simulink model "LFPCaseStudy_ZahidSarigol"  (R2025b)
settings: Solver=VariableStepAuto  StartTime=0.0  StopTime=3600  RelTol=1e-3
libraries: fl_lib x5, nesl_utility x3, batt_lib x1
settings Model: Creator=zahid  LastModifiedBy=zahid

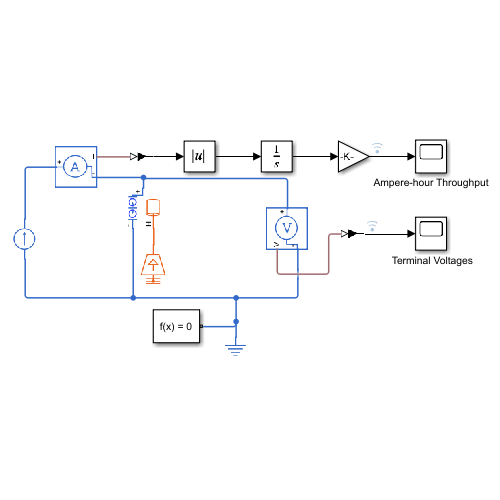
[thumbnail: Simulink's stored preview of the top-level diagram]
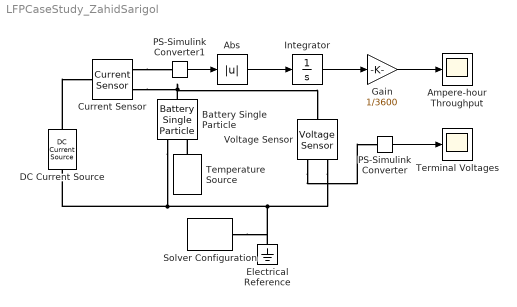
== system LFPCaseStudy_ZahidSarigol ==
  " Terminal Voltages" : Scope
      settings: ActiveDisplayYMinimum=2.7369582029139718  ActiveDisplayYMaximum=3.8258448981690734  YLabel=Voltage (V)
  Abs : Abs  SaturateOnIntegerOverflow=off
  Ampere-hour Throughput : Scope
      settings: ActiveDisplayYMinimum=-0.26295274335598895  ActiveDisplayYMaximum=2.3665746902039011  YLabel=Capacity (Ah)
  Battery Single Particle : batt_lib/Cells/Electrochemical/Battery Single Particle  ExtrapolationMethod=simscape.enum.extrapolation.nearest  ThicknessAnode=3.4E-5 m  ElectrolyteLayerCountAnode=10  ThicknessSeparator=2.5E-5 m  ElectrolyteLayerCountSeparator=5  ThicknessCathode=8E-5 m  ElectrolyteLayerCountCathode=10  ElectrodePlateArea=1.738E-1 m^2  ParticleRadiusAnode=3.5E-6 m  ShellCountAnode=10  ParticleRadiusCathode=5.2E-8 m  ShellCountCathode=10  ActiveMaterialVolumeFractionAnode=0.56  ActiveMaterialVolumeFractionCathode=0.454  StoichiometryBreakpointsSpecification=simscape.battery.enum.cells.electrochemical.StoichiometryBreakpointsSpecification.normalized  NormalizedStoichiometryBreakpoints=linspace(0.025, 0.975, 39)  OpenCircuitPotentialAnode=[.484; .335; .253; .209; .2; .181; .165; .151; .139; .131; .128; .125; .124; .124; .123; .122; .119; .117; .111; .108; .101; .098; .095; .093; .092; .088; .088; .088; .088; .087; .087; .087; .085; .082; .079; .071; .064; .049; .026] V  OpenCircuitPotentialCathode=[3.81;3.608;3.512;3.478;3.459;3.453;3.45257;3.45214;3.45171;3.45128;3.45085;3.45042;3.44999;3.44956;3.44913;3.4487;3.44827;3.44784;3.44741;3.44698;3.44655;3.44612;3.44569;3.44526;3.44483;3.4444;3.44397;3.44354;3.44311;3.44268;3.44225;3.44182;3.44139;3.44096;3.44053;3.44;3.412;3.304;2.968] V  AbsoluteStoichiometryBreakpointsAnode=linspace(0.025, 0.975, 39)  OpenCircuitPotentialAbsoluteAnode=[.484; .335; .253; .209; .2; .181; .165; .151; .139; .131; .128; .125; .124; .124; .123; .122; .119; .117; .111; .108; .101; .098; .095; .093; .092; .088; .088; .088; .088; .087; .087; .087; .085; .082; .079; .071; .064; .049; .026] V  AbsoluteStoichiometryBreakpointsCathode=linspace(0.025, 0.975, 39)  OpenCircuitPotentialAbsoluteCathode=[3.81; 3.608; 3.512; 3.478; 3.459; 3.453; 3.45257; 3.45214; 3.45171; 3.45128; 3.45085; 3.45042; 3.44999; 3.44956; 3.44913; 3.4487; 3.44827; 3.44784; 3.44741; 3.44698; 3.44655; 3.44612; 3.44569; 3.44526; 3.44483; 3.4444; 3.44397; 3.44354; 3.44311; 3.44268; 3.44225; 3.44182; 3.44139; 3.44096; 3.44053; 3.44; 3.412; 3.304; 2.968] V  MaximumConcentrationAnode=31900 mol/m^3  MaximumStoichiometryAnode=0.811  MinimumStoichiometryAnode=0.0132  MaximumConcentrationCathode=20950 mol/m^3  MaximumStoichiometryCathode=0.74  MinimumStoichiometryCathode=0.035  ActiveMaterialDiffusionCoefficientAnode=3E-15 m^2/s  ActiveMaterialDiffusionCoefficientCathode=8E-18 m^2/s  ConductivityAnode=200 S/m  ConductivityCathode=0.1 S/m  CurrentCollectorResistance=0 Ohm  ElectrolyteVolumeFractionAnode=0.3874  ElectrolyteVolumeFractionSeparator=0.45  ElectrolyteVolumeFractionCathode=0.5725  ElectrolyteConductivity=0.29 S/m  BruggemanExponentAnode=1.5  BruggemanExponentSeparator=1.5  BruggemanExponentCathode=1.5  TransferenceNumber=0.363  ElectrolyteDiffusionCoefficient=2E-10 m^2/s  ChargeTransferRateAnode=8.8E-11 m^(5/2)/(mol^(1/2)*s)  ChargeTransferRateCathode=2.8E-13 m^(5/2)/(mol^(1/2)*s)  BatteryThermalMass=77 J/K  ArrheniusReferenceTemperature=298.15 K  ActiveMaterialDiffusionActivationEnergyAnode=39000 J/mol  ActiveMaterialDiffusionActivationEnergyCathode=35000 J/mol  ElectrolyteDiffusionActivationEnergy=26600 J/mol  ConductivityActivationEnergyAnode=3000 J/mol  ConductivityActivationEnergyCathode=3000 J/mol  ElectrolyteConductivityActivationEnergy=11000 J/mol  ChargeTransferActivationEnergyAnode=13000 J/mol  ChargeTransferActivationEnergyCathode=20000 J/mol  batteryCurrent_specify=off  batteryCurrent_priority=None  batteryCurrent=0 A  batteryCurrent_nominal_specify=off  batteryCurrent_nominal_value=1  batteryCurrent_nominal_unit=A  batteryVoltage_specify=off  batteryVoltage_priority=None  batteryVoltage=0 V  batteryVoltage_nominal_specify=off  batteryVoltage_nominal_value=1  batteryVoltage_nominal_unit=V  averageElectrolyteConcentration_specify=off  averageElectrolyteConcentration_priority=High  averageElectrolyteConcentration=1200 mol/m^3  averageElectrolyteConcentration_nominal_specify=off  averageElectrolyteConcentration_nominal_value=1  averageElectrolyteConcentration_nominal_unit=mol/m^3  stateOfCharge_specify=on  stateOfCharge_priority=High  stateOfCharge=1  stateOfCharge_nominal_specify=off  stateOfCharge_nominal_value=1  stateOfCharge_nominal_unit=1  batteryTemperature_specify=off  batteryTemperature_priority=High  batteryTemperature=298.15 K  batteryTemperature_nominal_specify=off  batteryTemperature_nominal_value=1  batteryTemperature_nominal_unit=K  power_dissipated_specify=off  power_dissipated_priority=None  power_dissipated=0 W  power_dissipated_nominal_specify=off  power_dissipated_nominal_value=1  power_dissipated_nominal_unit=W  heatGenerationRate_specify=off  heatGenerationRate_priority=None  heatGenerationRate=0 W  heatGenerationRate_nominal_specify=off  heatGenerationRate_nominal_value=1  heatGenerationRate_nominal_unit=W
      settings: InternalSimscapePortConfiguration="{\"Bottom\":[],\"Left\":[{\"id\":\"p\",\"label\":\"+\",\"type\":\"foundation.electrical.electrical\"}],\"Right\":[{\"id\":\"n\",\"label\":\"-\",\"type\":\"foundation.electrical.electrical\"},{\"id\":\"H\",\"label\":\"H\",\"type\":\"foundation.thermal.thermal\"}],\"Top\":[]}"
  Current Sensor : fl_lib/Electrical/Electrical Sensors/Current Sensor
  DC Current Source : fl_lib/Electrical/Electrical Sources/DC Current Source  i0=-2.5 A
      settings: InternalSimscapePortConfiguration="{\"Bottom\":[],\"Left\":[{\"id\":\"p\",\"label\":\"\",\"type\":\"foundation.electrical.electrical\"}],\"Right\":[{\"id\":\"n\",\"label\":\"\",\"type\":\"foundation.electrical.electrical\"}],\"Top\":[]}"
  Electrical Reference : fl_lib/Electrical/Electrical Elements/Electrical Reference
  Gain : Gain  Gain=1/3600
  Integrator : Integrator
  PS-Simulink Converter : nesl_utility/PS-Simulink Converter  PhysicalDomain=network_engine_domain  SubClassName=ps_output  LeftPortType=input  RightPortType=output  PseudoPeriodic=off  Frequencies=[]  VectorFormat=inherit  Unit=inherit  AffineConversion=off
  PS-Simulink Converter1 : nesl_utility/PS-Simulink Converter  PhysicalDomain=network_engine_domain  SubClassName=ps_output  LeftPortType=input  RightPortType=output  PseudoPeriodic=off  Frequencies=[]  VectorFormat=inherit  Unit=inherit  AffineConversion=off
  Solver Configuration : nesl_utility/Solver Configuration  PhysicalDomain=network_engine_domain  SubClassName=solver  LeftPortType=input  RightPortType=generic  Tones=[]  Harmonics=[]  SimulateNoise=off  Profile=off  UseLocalSampling=off  EnableSwitchedLinearOptims=on  FrequencyDomain=off  UseCCode=off  RelTol=0.001  AbsTol=0.001  MinStep=1e-09  ToWorkspace=off  RevertToSquareIcSolve=off  NumHomotopyIterations=100  PhasorMode=off  PhasorModeNumHarmonics=1  ConsistencySolver=NEWTON_XTOL_AFTER_FTOL  IndexReductionMethod=DerivativeReplacement  DoDC=off  ResidualTolerance=1e-09  ConsistencyTolSource=GLOBAL  ConsistencyAbsTol=0.001  ConsistencyRelTol=0.001  ConsistencyTolFactor=0.001  UseLocalSolver=off  LocalSolverChoice=NE_BACKWARD_EULER_ADVANCER  ResolveIndetEquations=on  FunctionEvalNumThread=1  LocalSolverSampleTime=0.001  DoFixedCost=off  MaxNonlinIter=3  MaxModeIter=2  ComputeImpulses=off  ImpulseIterations=2  LinearAlgebra=auto  LinearAlgebraNumThread=0  EquationFormulation=NE_TIME_EF  DelaysMemoryBudget=1024  AutomaticFiltering=on  FilteringTimeConstant=0.001  PartitionStorageMethod=AS_NEEDED  PartitionMemoryBudget=1024  PartitionMethod=ROBUST  MultibodyUseLocalSolver=off  MultibodyLocalSolverChoice=ODE1  MultibodyLocalSolverSampleTime=0.001
  Temperature Source : fl_lib/Thermal/Thermal Sources/Temperature Source  temperature=298.15 K
  Voltage Sensor : fl_lib/Electrical/Electrical Sensors/Voltage Sensor
  wires:
  PS-Simulink Converter/1 -> " Terminal Voltages"/1
  PS-Simulink Converter1/1 -> Abs/1
  Abs/1 -> Integrator/1
  Integrator/1 -> Gain/1
  Gain/1 -> Ampere-hour Throughput/1
  connections:
  Temperature Source/LConn1 -- Battery Single Particle/RConn2
  Battery Single Particle/LConn1 -- Voltage Sensor/LConn1 -- Current Sensor/RConn2
  Battery Single Particle/RConn1 -- Voltage Sensor/RConn2 -- Solver Configuration/RConn1 -- Electrical Reference/LConn1 -- DC Current Source/RConn1
  Voltage Sensor/RConn1 -- PS-Simulink Converter/LConn1
  DC Current Source/LConn1 -- Current Sensor/LConn1
  Current Sensor/RConn1 -- PS-Simulink Converter1/LConn1
